simulink model "gm_majorChangeShift"  (R2022a)
settings: Solver=VariableStepAuto  StartTime=0.0  StopTime=3  RelTol=1e-3
PostLoadFcn:
  | postLoadCallback
InitFcn:
  | initCallback
StopFcn:
  | stopCallback
undefined symbols (not defined in the file or in its folder): modelParams
libraries: hdlsllib x8, dspsrcs4 x3
settings Model: Creator=Ronnel  LastModifiedBy=Ronnel
settings DataIOCC: ReturnWorkspaceOutputs=off
settings OptimizationCC: BlockReduction=off  ConditionallyExecuteInputs=off  DefaultParameterBehavior=Inlined
settings DebuggingCC: AlgebraicLoopMsg=error  InheritedTsInSrcMsg=none
settings HardwareCC: ProdBitPerPointer=32  ProdBitPerSizeT=32  ProdBitPerPtrDiffT=32  ProdLargestAtomicFloat=None  ProdIntDivRoundTo=Undefined  ProdEndianess=Unspecified  ProdWordSize=32  ProdHWDeviceType=ASIC/FPGA->ASIC/FPGA  TargetBitPerPointer=64  TargetBitPerSizeT=64  TargetBitPerPtrDiffT=64  TargetLongLongMode=on  TargetIntDivRoundTo=Zero  TargetEndianess=LittleEndian  TargetWordSize=64  TargetHWDeviceType=Custom Processor->MATLAB Host Computer  ProdEqTarget=off

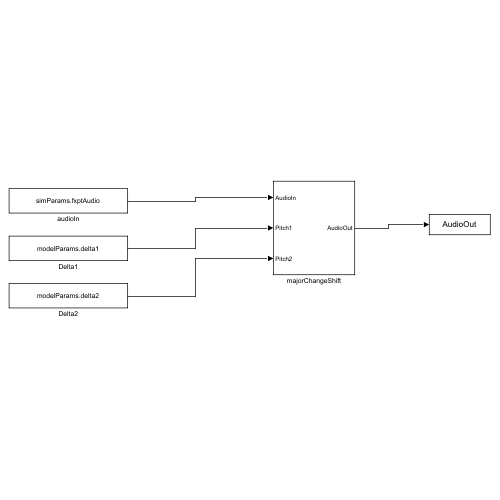
[thumbnail: Simulink's stored preview of the top-level diagram]
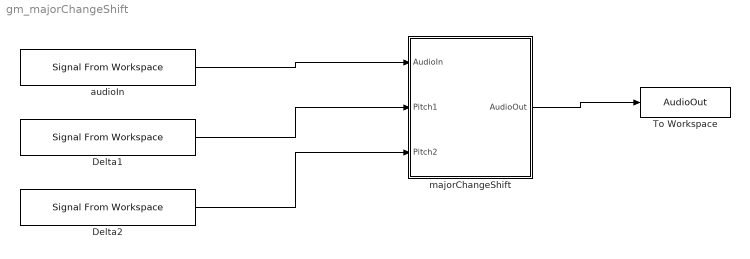
== system gm_majorChangeShift ==
  Delta1 : dspsrcs4/Signal From Workspace  X=modelParams.delta1  Ts=modelParams.audio.samplePeriod  nsamps=1  OutputAfterFinalValue=Setting to zero  ignoreOrWarnInputAndFrameLengths=off  OutputFrames=off
  Delta2 : dspsrcs4/Signal From Workspace  X=modelParams.delta2  Ts=modelParams.audio.samplePeriod  nsamps=1  OutputAfterFinalValue=Setting to zero  ignoreOrWarnInputAndFrameLengths=off  OutputFrames=off
  To Workspace : ToWorkspace  VariableName=AudioOut  SampleTime=-1
      settings: Save2DSignal=2-D array (concatenate along first dimension)
  audioIn : dspsrcs4/Signal From Workspace  X=simParams.fxptAudio  Ts=modelParams.audio.samplePeriod  nsamps=1  OutputAfterFinalValue=Setting to zero  ignoreOrWarnInputAndFrameLengths=off  OutputFrames=off
  majorChangeShift : Subsystem
  wires:
  Delta2/1 -> majorChangeShift/3(Pitch2)
  Delta1/1 -> majorChangeShift/2(Pitch1)
  majorChangeShift/1(AudioOut) -> To Workspace/1
  audioIn/1 -> majorChangeShift/1(AudioIn)

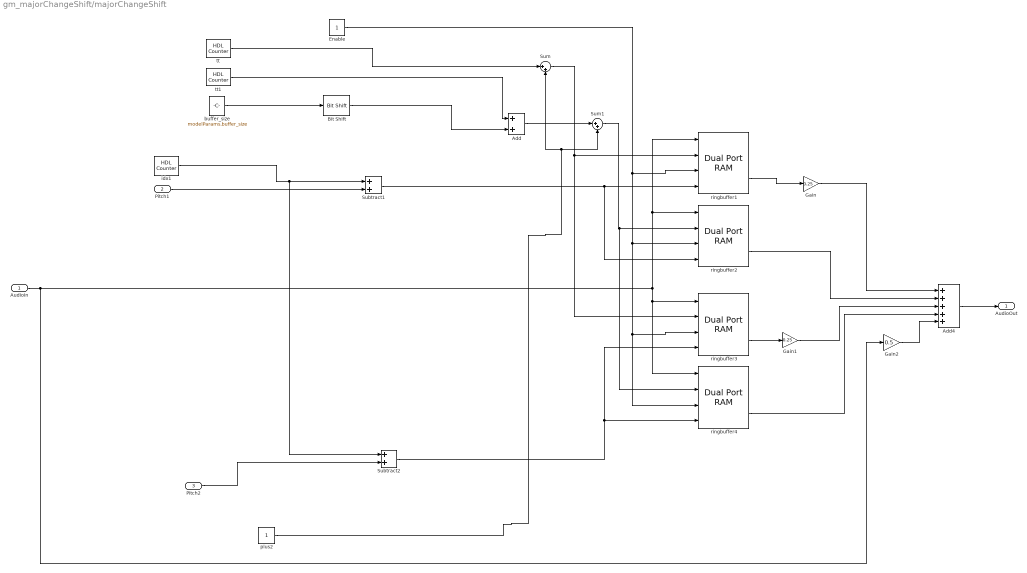
== system gm_majorChangeShift/majorChangeShift ==
  AudioIn : Inport  SampleTime=modelParams.audio.samplePeriod
  Pitch1 : Inport  Port=2  SampleTime=modelParams.audio.samplePeriod
  Pitch2 : Inport  Port=3  SampleTime=modelParams.audio.samplePeriod
  Add : Sum  SampleTime=modelParams.audio.samplePeriod
  Add4 : Sum  Inputs=+++++  OutDataTypeStr=fixdt(1,24,16)  SampleTime=modelParams.audio.samplePeriod
  Bit Shift : hdlsllib/Logic and Bit Operations/Bit Shift  mode=Shift Right Logical  N=1
  Enable : Constant  OutDataTypeStr=boolean  SampleTime=modelParams.audio.samplePeriod
  Gain : Gain  Gain=0.25  SampleTime=modelParams.audio.samplePeriod
  Gain1 : Gain  Gain=0.25  SampleTime=modelParams.audio.samplePeriod
  Gain2 : Gain  Gain=0.5  SampleTime=modelParams.audio.samplePeriod
  Subtract1 : Sum  OutDataTypeStr=Inherit: Inherit via back propagation  RndMeth=Round  SampleTime=modelParams.audio.samplePeriod
  Subtract2 : Sum  OutDataTypeStr=Inherit: Inherit via back propagation  RndMeth=Round  SampleTime=modelParams.audio.samplePeriod
  Sum : Sum  Inputs=|++  OutDataTypeStr=uint16  SampleTime=modelParams.audio.samplePeriod
  Sum1 : Sum  Inputs=|++  OutDataTypeStr=uint16  SampleTime=modelParams.audio.samplePeriod
  buffer_size : Constant  Value=modelParams.buffer_size  SampleTime=modelParams.audio.samplePeriod
  idx1 : hdlsllib/Sources/HDL Counter  CountType=Free running  CountInit=0  CountStep=1  CountMax=25  CountFromType=Initial value  CountFrom=0  CountResetPort=off  CountLoadPort=off  CountEnbPort=off  CountDirPort=off  CountHitOutputPort=off  CountDataType=Unsigned  CountWordLen=modelParams.dpramAddressSize + modelParams.audio.fractionLength  CountFracLen=modelParams.audio.fractionLength  CountSampTime=modelParams.audio.samplePeriod
  plus2 : Constant  OutDataTypeStr=Inherit: Inherit via back propagation  SampleTime=modelParams.audio.samplePeriod
  ringbuffer{1..4} (4 alike) : hdlsllib/HDL RAMs/Dual Port RAM  ram_size=16
      settings: SourceProductBaseCode=SL
  tt : hdlsllib/Sources/HDL Counter  CountType=Free running  CountInit=1  CountStep=1  CountMax=25  CountFromType=Initial value  CountFrom=1  CountResetPort=off  CountLoadPort=off  CountEnbPort=off  CountDirPort=off  CountHitOutputPort=off  CountDataType=Unsigned  CountWordLen=modelParams.dpramAddressSize  CountFracLen=0  CountSampTime=modelParams.audio.samplePeriod
  tt1 : hdlsllib/Sources/HDL Counter  CountType=Free running  CountInit=1  CountStep=1  CountMax=25  CountFromType=Initial value  CountFrom=1  CountResetPort=off  CountLoadPort=off  CountEnbPort=off  CountDirPort=off  CountHitOutputPort=off  CountDataType=Unsigned  CountWordLen=modelParams.dpramAddressSize-1  CountFracLen=0  CountSampTime=modelParams.audio.samplePeriod
  AudioOut : Outport
  wires:
  Gain2/1 -> Add4/5
  AudioIn/1 -> Gain2/1, ringbuffer1/1, ringbuffer2/1, ringbuffer3/1, ringbuffer4/1
  Enable/1 -> ringbuffer1/3, ringbuffer2/3, ringbuffer3/3, ringbuffer4/3
  ringbuffer4/2 -> Add4/4
  Pitch2/1 -> Subtract2/2
  Sum1/1 -> ringbuffer2/2, ringbuffer4/2
  Bit Shift/1 -> Add/2
  Sum/1 -> ringbuffer1/2, ringbuffer3/2
  ringbuffer3/2 -> Gain1/1
  Subtract2/1 -> ringbuffer4/4, ringbuffer3/4
  Gain1/1 -> Add4/3
  idx1/1 -> Subtract1/1, Subtract2/1
  Pitch1/1 -> Subtract1/2
  tt1/1 -> Add/1
  Add4/1 -> AudioOut/1
  Subtract1/1 -> ringbuffer2/4, ringbuffer1/4
  plus2/1 -> Sum1/2, Sum/2
  Gain/1 -> Add4/1
  tt/1 -> Sum/1
  ringbuffer1/2 -> Gain/1
  buffer_size/1 -> Bit Shift/1
  Add/1 -> Sum1/1
  ringbuffer2/2 -> Add4/2
